simulink model "Regenerative_Braking"  (R2023a)
settings: Solver=ode23tb  StartTime=0.0  StopTime=300  MaxStep=0.1  MinStep=1e-4  RelTol=1e-2
values from neighbouring files (symbols this model uses):
  SOC = simOut.get('SOC')    [untitled.m]
undefined symbols (not defined in the file or in its folder): canChannel, T_cell
libraries: canmsglib x6, simulink x4, canlib x1
settings Model: Creator=MEHMET  LastModifiedBy=MEHMET
settings SolverCC: MaxConsecutiveMinStep=20
settings DebuggingCC: AlgebraicLoopMsg=none  ArtificialAlgebraicLoopMsg=none  ParameterPrecisionLossMsg=none  OperatingPointInterfaceChecksumMismatchMsg=none

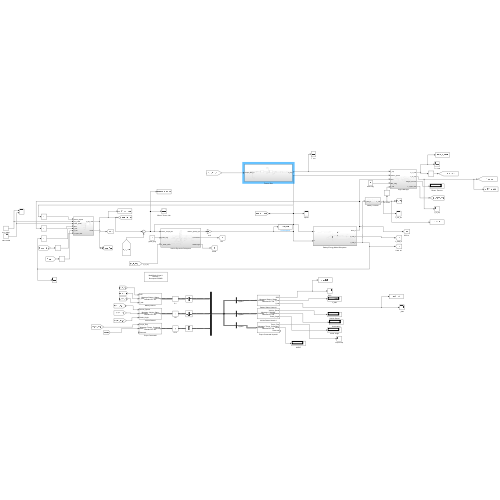
[thumbnail: Simulink's stored preview of the top-level diagram]
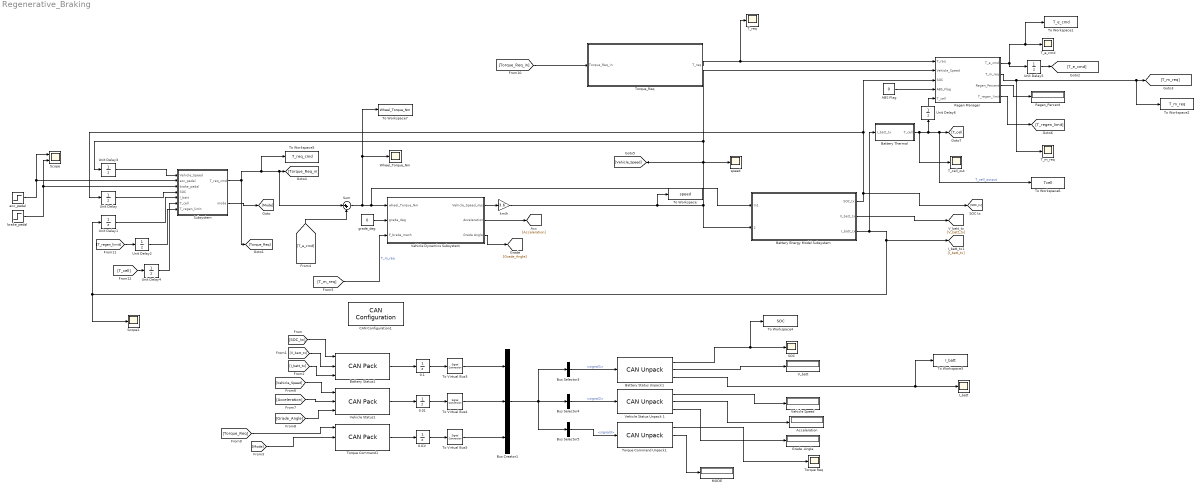
== system Regenerative_Braking ==
  0.01 : UnitDelay  InitialCondition=0.01  SampleTime=-1  HasFrameUpgradeWarning=on
  0.01! : UnitDelay  InitialCondition=0.1  SampleTime=-1  HasFrameUpgradeWarning=on
  0.1 : UnitDelay  InitialCondition=0.1  SampleTime=-1  HasFrameUpgradeWarning=on
  ABS Flag : Constant  Value=0
  Acceleration : Display
  Battery Energy Model Subsystem : Subsystem
  Battery Status Unpack1 : canmsglib/CAN Unpack  MsgList=(none)  MsgName=Battery_Status  MsgIDType=Standard (11-bit identifier)  MsgIdentifier=100  MsgLength=8  SignalInfo={ 'SOC', '0', '16', 'LE', 'signed', 'Standard', '0', '0.1', '0', '-Inf', 'Inf'; 'V_batt', '16', '16', 'LE', 'unsigned', 'Standard', '0', '0.1', '0', '-Inf', 'Inf'; 'I_batt', '32', '16', 'LE', 'signed', 'Standard', '0', '0.01', '0', '-Inf', 'Inf' }  IDPort=off  TimestampPort=off  ErrorPort=off  RemotePort=off  LengthPort=off  StatusPort=off  ApplyMinMax=off
      settings: LibrarySourceBlock=canlib/CAN Unpack
  Battery Status1 : canmsglib/CAN Pack  MsgList=(none)  MsgName=Battery_Status  MsgIDType=Standard (11-bit identifier)  MsgIdentifier=100  MsgLength=8  Remote=off  ApplyMinMax=off  BusOutput=on  SignalInfo={ 'SOC', '0', '16', 'LE', 'signed', 'Standard', '0', '0.1', '0', '-Inf', 'Inf'; 'V_batt', '16', '16', 'LE', 'unsigned', 'Standard', '0', '0.1', '0', '-Inf', 'Inf'; 'I_batt', '32', '16', 'LE', 'signed', 'Standard', '0', '0.01', '0', '-Inf', 'Inf' }
      settings: LibrarySourceBlock=canlib/CAN Pack  DataFormat=manually specified signals
  Battery Thermal : Subsystem
  Bus Creator1 : BusCreator  Inputs=3
  Bus Selector3 : BusSelector  OutputSignals=signal1
  Bus Selector4 : BusSelector  OutputSignals=signal2
  Bus Selector5 : BusSelector  OutputSignals=signal3
  CAN Configuration1 : canlib/CAN Configuration  BlockHandle=109.0284  Device=MathWorks Virtual 1 (Channel 1)  DeviceMenu=MathWorks Virtual 1 (Channel 1)  ObjConstructor=canChannel('MathWorks', 'Virtual 1', 1)  BusSpeed=500000  EnableBitParameters=off  AckMode=Normal
  Grade .Angle : Display
  I_batt : Scope
  MODE : Display
  Regen Manager : Subsystem
  Regen_Percent : Display
  SOC : Scope
  Scope : Scope  NumInputPorts=2
  Scope1 : Scope
  Subsystem : Subsystem
  Sum : Sum  Inputs=|++
  T_cell_out : Scope
  T_e_cmd : Scope
  T_m_req : Scope
  T_req : Scope
  To Virtual Bus3 : SignalConversion  ConversionOutput=Nonvirtual bus  OverrideOpt=off
  To Virtual Bus4 : SignalConversion  ConversionOutput=Nonvirtual bus  OverrideOpt=off
  To Virtual Bus5 : SignalConversion  ConversionOutput=Nonvirtual bus  OverrideOpt=off
  To Workspace : ToWorkspace  VariableName=speed  SampleTime=-1
  To Workspace1 : ToWorkspace  VariableName=T_e_cmd  SampleTime=-1
  To Workspace2 : ToWorkspace  VariableName=T_m_req  SampleTime=-1
  To Workspace3 : ToWorkspace  VariableName=I_batt  SampleTime=-1
  To Workspace4 : ToWorkspace  VariableName=SOC  SampleTime=-1
  To Workspace5 : ToWorkspace  VariableName=T_req_cmd  SampleTime=-1
  To Workspace6 : ToWorkspace  VariableName=Tcell  SampleTime=-1
  To Workspace7 : ToWorkspace  VariableName=Wheel_Torque_Nm  SampleTime=-1
  Torque Command Unpack1 : canmsglib/CAN Unpack  MsgList=(none)  MsgName=Torque_Command  MsgIDType=Standard (11-bit identifier)  MsgIdentifier=300  MsgLength=8  SignalInfo={ 'Torque_Req', '0', '32', 'LE', 'single', 'Standard', '0', '1', '0', '-Inf', 'Inf'; 'Mode', '32', '8', 'LE', 'unsigned', 'Standard', '0', '1', '0', '-Inf', 'Inf'; 'Reserved', '40', '8', 'LE', 'unsigned', 'Standard', '0', '1', '0', '-Inf', 'Inf' }  IDPort=off  TimestampPort=off  ErrorPort=off  RemotePort=off  LengthPort=off  StatusPort=off  ApplyMinMax=off
      settings: LibrarySourceBlock=canlib/CAN Unpack
  Torque Command1 : canmsglib/CAN Pack  MsgList=(none)  MsgName=Torque_Command  MsgIDType=Standard (11-bit identifier)  MsgIdentifier=300  MsgLength=8  Remote=off  ApplyMinMax=off  BusOutput=on  SignalInfo={ 'Torque_Req', '0', '32', 'LE', 'single', 'Standard', '0', '1', '0', '-Inf', 'Inf'; 'Mode', '32', '8', 'LE', 'unsigned', 'Standard', '0', '1', '0', '-Inf', 'Inf'; 'Reserved', '40', '8', 'LE', 'unsigned', 'Standard', '0', '1', '0', '-Inf', 'Inf' }
      settings: LibrarySourceBlock=canlib/CAN Pack  DataFormat=manually specified signals
  Torque Req : Scope
  Torque_Req : Subsystem
  Unit Delay{,1..5} (6 alike) : UnitDelay  SampleTime=0.01  HasFrameUpgradeWarning=on
  Unit Delay6 : UnitDelay  InitialCondition=0.01  SampleTime=-1  HasFrameUpgradeWarning=on
  V_batt : Display
  Vehicle Dynamics Subsystem : Subsystem
  Vehicle Speed : Display
  Vehicle Status Unpack 1 : canmsglib/CAN Unpack  MsgList=(none)  MsgName=CAN Msg  MsgIDType=Standard (11-bit identifier)  MsgIdentifier=200  MsgLength=8  SignalInfo={ 'Vehicle_Speed', '0', '16', 'LE', 'unsigned', 'Standard', '0', '0.1', '0', '-Inf', 'Inf'; 'Acceleration', '16', '16', 'LE', 'unsigned', 'Standard', '0', '0.01', '0', '-Inf', 'Inf'; 'Grade_Angle', '32', '16', 'LE', 'unsigned', 'Standard', '0', '0.1', '0', '-Inf', 'Inf' }  IDPort=off  TimestampPort=off  ErrorPort=off  RemotePort=off  LengthPort=off  StatusPort=off  ApplyMinMax=off
      settings: LibrarySourceBlock=canlib/CAN Unpack
  Vehicle Status1 : canmsglib/CAN Pack  MsgList=(none)  MsgName=Vehicle_State  MsgIDType=Standard (11-bit identifier)  MsgIdentifier=200  MsgLength=8  Remote=off  ApplyMinMax=off  BusOutput=on  SignalInfo={ 'Vehicle_Speed', '0', '16', 'LE', 'unsigned', 'Standard', '0', '0.1', '0', '-Inf', 'Inf'; 'Acceleration', '16', '16', 'LE', 'unsigned', 'Standard', '0', '0.01', '0', '-Inf', 'Inf'; 'Grade_Angle', '32', '16', 'LE', 'unsigned', 'Standard', '0', '0.1', '0', '-Inf', 'Inf' }
      settings: LibrarySourceBlock=canlib/CAN Pack  DataFormat=manually specified signals
  Wheel_Torque_Nm : Scope
  acc_pedal : Step  After=100  SampleTime=0  ZeroCross=off
  brake_pedal : Step  Time=100  After=300  SampleTime=0  ZeroCross=off
  grade_deg : Constant  Value=0
  km/h : Gain  Gain=3.6
  speed : Scope
  wires:
  Regen Manager/1(T_e_cmd) -> Unit Delay5/1, To Workspace1/1, T_e_cmd/1
  [Acceleration] -> Vehicle Status1/2
  Vehicle Status Unpack 1/2 -> Acceleration/1
  Vehicle Dynamics Subsystem/1(Vehicle_Speed_mps) -> km/h/1
  [Vehicle_Speed] -> Vehicle Status1/1
  Bus Creator1/1 -> Bus Selector5/1, Bus Selector3/1, Bus Selector4/1
  [Mode] -> Torque Command1/2
  Battery Status Unpack1/1 -> To Workspace4/1, SOC/1
  Battery Status Unpack1/3 -> To Workspace3/1, I_batt/1
  Battery Status Unpack1/2 -> V_batt/1
  [I_batt_tx] -> Battery Status1/3
  Bus Selector3/1 -> Battery Status Unpack1/1  "<signal1>"
  Vehicle Status Unpack 1/3 -> Grade .Angle/1
  Bus Selector4/1 -> Vehicle Status Unpack 1/1  "<signal2>"
  To Virtual Bus3/1 -> Bus Creator1/1
  Bus Selector5/1 -> Torque Command Unpack1/1  "<signal3>"
  Torque Command Unpack1/2 -> MODE/1
  Battery Status1/1 -> 0.1/1
  To Virtual Bus5/1 -> Bus Creator1/3
  Vehicle Dynamics Subsystem/3(Grade Angle) -> [Grade_Angle]
  To Virtual Bus4/1 -> Bus Creator1/2
  [V_batt_tx] -> Battery Status1/2
  Battery Energy Model Subsystem/2(V_batt_tx) -> [V_batt_tx]
  [SOC_tx] -> Battery Status1/1
  Vehicle Dynamics Subsystem/2(Acceleration) -> [Acceleration]
  [Grade_Angle] -> Vehicle Status1/3
  Regen Manager/3(Regen_Percent) -> Regen_Percent/1
  Torque Command1/1 -> 0.01!/1
  Regen Manager/2(T_m_req) -> T_m_req/1, To Workspace2/1, [T_m_req]
  grade_deg/1 -> Vehicle Dynamics Subsystem/2(grade_deg)
  0.01!/1 -> To Virtual Bus5/1
  ABS Flag/1 -> Regen Manager/4(ABS_Flag)
  Vehicle Status1/1 -> 0.01/1
  Torque Command Unpack1/1 -> Torque Req/1
  0.1/1 -> To Virtual Bus3/1
  Vehicle Status Unpack 1/1 -> Vehicle Speed/1
  Battery Energy Model Subsystem/3(I_batt_tx) -> Scope1/1, Unit Delay1/1, [I_batt_tx], Battery Thermal/1(I_batt_tx)
  [Torque_Req] -> Torque Command1/1
  Torque_Req/1(T_req) -> T_req/1, Regen Manager/1(T_req)
  0.01/1 -> To Virtual Bus4/1
  [Torque_Req_in] -> Torque_Req/1(Torque_Req_in)
  Sum/1 -> To Workspace7/1, Wheel_Torque_Nm/1, Battery Energy Model Subsystem/1(In1), Vehicle Dynamics Subsystem/1(wheel_Torque_Nm)
  [T_e_cmd] -> Sum/2
  [T_m_req] -> Vehicle Dynamics Subsystem/3(F_brake_mech)  "T_m_req"
  km/h/1 -> To Workspace/1, Unit Delay3/1, Regen Manager/2(Vehicle_Speed), speed/1, [Vehicle_Speed], Battery Energy Model Subsystem/2(2)
  Battery Energy Model Subsystem/1(SOC_tx) -> [SOC_tx], Regen Manager/3(SOC), Unit Delay/1
  Regen Manager/4(T_regen_limit) -> [T_regen_limit]
  Battery Thermal/1(T_cell) -> Unit Delay6/1, To Workspace6/1, [T_cell], T_cell_out/1  "T_cell_output"
  [T_regen_limit] -> Unit Delay2/1
  [T_cell] -> Unit Delay4/1
  Unit Delay5/1 -> [T_e_cmd]
  Unit Delay6/1 -> Regen Manager/5(T_cell)
  acc_pedal/1 -> Subsystem/2(acc_pedal), Scope/1
  brake_pedal/1 -> Subsystem/3(brake_pedal), Scope/2
  Unit Delay3/1 -> Subsystem/1(Vehicle_Speed)
  Unit Delay/1 -> Subsystem/4(SOC)
  Unit Delay1/1 -> Subsystem/5(I_batt)
  Unit Delay4/1 -> Subsystem/6(T_cell)
  Unit Delay2/1 -> Subsystem/7(T_regen_limit)
  Subsystem/1(T_req_cmd) -> To Workspace5/1, Sum/1, [Torque_Req_in], [Torque_Req]
  Subsystem/2(mode) -> [Mode]

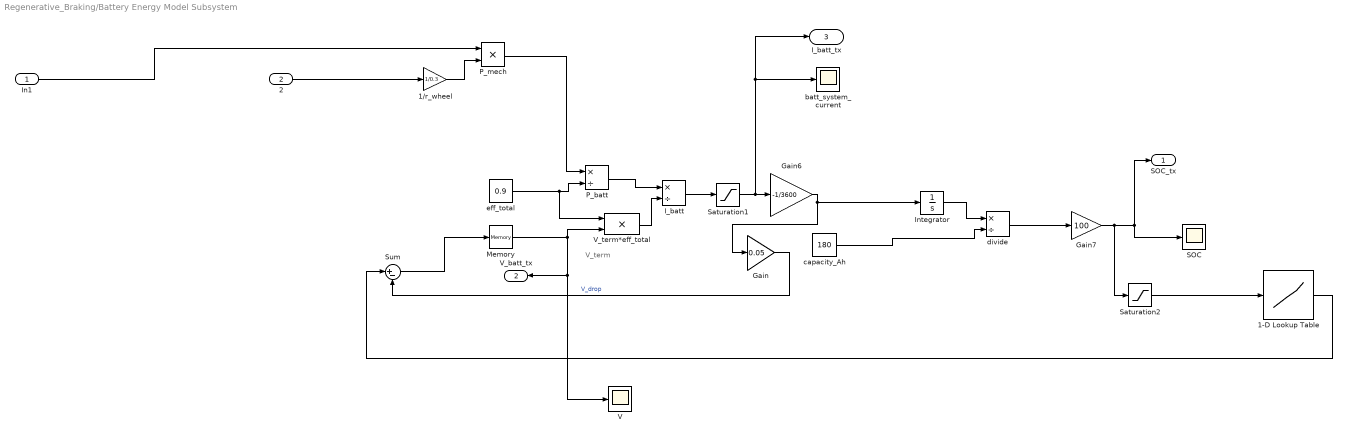
== system Regenerative_Braking/Battery Energy Model Subsystem ==
  note: V_term
  In1 : Inport
  2 : Inport  Port=2
  1-D Lookup Table : Lookup_n-D  NumberOfTableDimensions=1  BreakpointsForDimension1=[10 20 40 60 80 100]  Table=[325 332 342 350 356 360]  InternalRulePriority=Speed  RndMeth=Simplest
  1/r_wheel : Gain  Gain=1/0.3
  Gain : Gain  Gain=0.05
  Gain6 : Gain  Gain=-1/3600
  Gain7 : Gain  Gain=100
  I_batt : Product  Inputs=*/  RndMeth=Zero  SaturateOnIntegerOverflow=on
  Integrator : Integrator  InitialCondition=80  LimitOutput=on  UpperSaturationLimit=180  LowerSaturationLimit=0  ZeroCross=off
  Memory : Memory  InitialCondition=0.01
  P_batt : Product  Inputs=*/
  P_mech : Product
  SOC : Scope
  Saturation1 : Saturate  UpperLimit=300  LowerLimit=-300  ZeroCross=off
  Saturation2 : Saturate  UpperLimit=100  LowerLimit=0  ZeroCross=off
  Sum : Sum  Inputs=|+-
  V : Scope
  V_term*eff_total : Product
  batt_system_current : Scope
  capacity_Ah : Constant  Value=180
  divide : Product  Inputs=*/  RndMeth=Zero  SaturateOnIntegerOverflow=on
  eff_total : Constant  Value=0.9
  SOC_tx : Outport
  V_batt_tx : Outport  Port=2
  I_batt_tx : Outport  Port=3
  wires:
  P_batt/1 -> I_batt/1
  2/1 -> 1/r_wheel/1
  In1/1 -> P_mech/1
  capacity_Ah/1 -> divide/2
  1/r_wheel/1 -> P_mech/2
  P_mech/1 -> P_batt/1
  eff_total/1 -> V_term*eff_total/1, P_batt/2
  Gain7/1 -> Saturation2/1, SOC_tx/1, SOC/1
  1-D Lookup Table/1 -> Sum/1
  Memory/1 -> V/1, V_batt_tx/1, V_term*eff_total/2
  Sum/1 -> Memory/1
  Gain/1 -> Sum/2  "V_drop"
  V_term*eff_total/1 -> I_batt/2
  Integrator/1 -> divide/1
  I_batt/1 -> Saturation1/1
  Saturation1/1 -> I_batt_tx/1, batt_system_current/1, Gain6/1
  Saturation2/1 -> 1-D Lookup Table/1
  divide/1 -> Gain7/1
  Gain6/1 -> Integrator/1, Gain/1

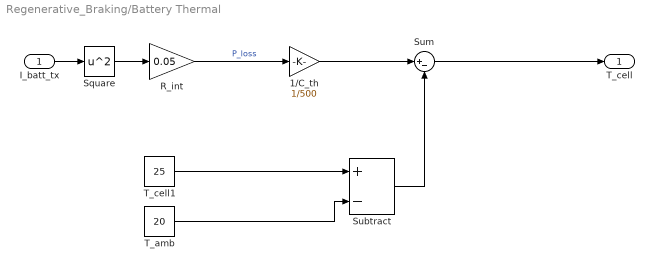
== system Regenerative_Braking/Battery Thermal ==
  I_batt_tx : Inport
  1/C_th : Gain  Gain=1/500
  R_int : Gain  Gain=0.05
  Square : Math  Operator=square
  Subtract : Sum  Inputs=+-
  Sum : Sum  Inputs=|+-
  T_amb : Constant  Value=20
  T_cell1 : Constant  Value=25
  T_cell : Outport
  wires:
  I_batt_tx/1 -> Square/1
  Square/1 -> R_int/1
  R_int/1 -> 1/C_th/1  "P_loss"
  1/C_th/1 -> Sum/1
  T_cell1/1 -> Subtract/1
  T_amb/1 -> Subtract/2
  Subtract/1 -> Sum/2
  Sum/1 -> T_cell/1

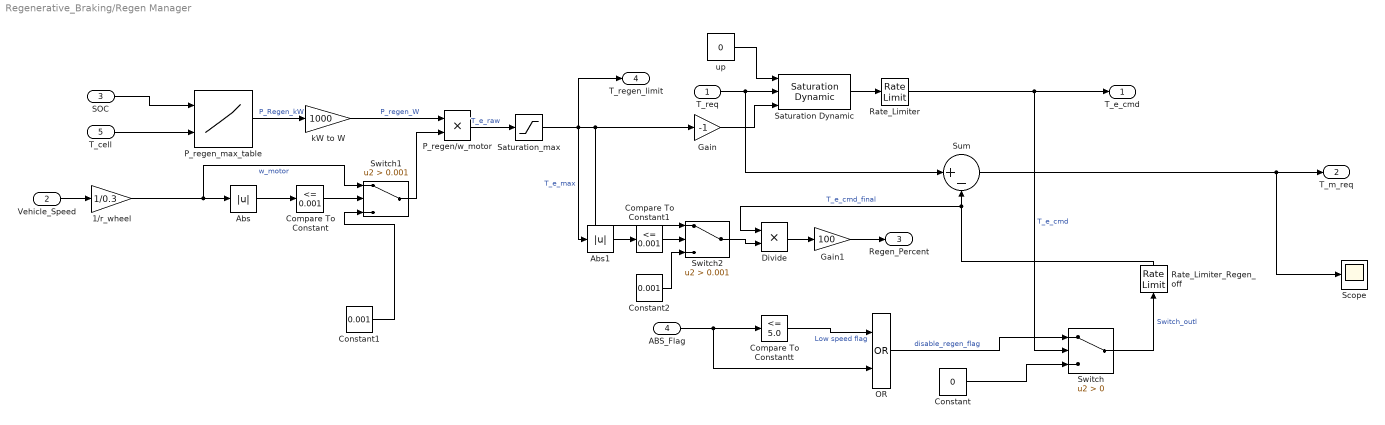
== system Regenerative_Braking/Regen Manager ==
  T_req : Inport
  Vehicle_Speed : Inport  Port=2
  SOC : Inport  Port=3
  ABS_Flag : Inport  Port=4
  T_cell : Inport  Port=5
  1/r_wheel : Gain  Gain=1/0.3
  Abs : Abs  ZeroCross=off  SaturateOnIntegerOverflow=off
  Abs1 : Abs  SaturateOnIntegerOverflow=off
  Compare To Constant : simulink/Logic and Bit Operations/Compare To Constant  relop=<=  const=0.001  OutDataTypeStr=boolean  ZeroCross=off
  Compare To Constant1 : simulink/Logic and Bit Operations/Compare To Constant  relop=<=  const=0.001  OutDataTypeStr=boolean  ZeroCross=off
  Compare To Constantt : simulink/Logic and Bit Operations/Compare To Constant  relop=<=  const=5.0  OutDataTypeStr=boolean  ZeroCross=off
  Constant : Constant  Value=0
  Constant1 : Constant  Value=0.001
  Constant2 : Constant  Value=0.001
  Divide : Product  RndMeth=Zero  SaturateOnIntegerOverflow=on
  Gain : Gain  Gain=-1
  Gain1 : Gain  Gain=100
  OR : Logic  Operator=OR  IconShape=distinctive  AllPortsSameDT=off  OutDataTypeStr=boolean
  P_regen/w_motor : Product  RndMeth=Zero  SaturateOnIntegerOverflow=on
  P_regen_max_table : Lookup_n-D  BreakpointsForDimension1=[0 20 40 60 80 95 100] % SOC  BreakpointsForDimension2="[-10 0 10 20 30 40 50]    % T_cell"  Table=|  InternalRulePriority=Speed  RndMeth=Simplest
      | [  5   10   15   20   25   20    0;
      |    8   15   25   35   45   35    0;
      |   12   30   45   60   70   50    0;
      |   15   40   60   80   90   60    0;
      |   15   40   60   80   90   60    0;
      |   10   30   45   60   70   50    0;
      |    5   15   25   35   45   35    0 ]
      settings: InputPortMap=u0,u1
  Rate_Limiter : RateLimiter  RisingSlewLimit=3000  FallingSlewLimit=-3000  SampleTimeMode=inherited
  Rate_Limiter_Regen_off : RateLimiter  RisingSlewLimit=2000  FallingSlewLimit=-2000  SampleTimeMode=inherited
  Saturation Dynamic : simulink/Discontinuities/Saturation Dynamic  OutMin=[]  OutMax=[]  OutDataTypeStr=Inherit: Same as second input  OutDataType=fixdt(1, 16)  OutScaling=2^-10  DoSatur=off
  Saturation_max : Saturate  UpperLimit=1500  LowerLimit=0  ZeroCross=off
  Scope : Scope
  Sum : Sum  Inputs=|+-
  Switch : Switch  Criteria=u2 > Threshold  SaturateOnIntegerOverflow=off  InputSameDT=off
  Switch1 : Switch  Criteria=u2 > Threshold  Threshold=0.001  SaturateOnIntegerOverflow=off  InputSameDT=off
  Switch2 : Switch  Criteria=u2 > Threshold  Threshold=0.001  SaturateOnIntegerOverflow=off  InputSameDT=off
  kW to W : Gain  Gain=1000
  up : Constant  Value=0
  T_e_cmd : Outport
  T_m_req : Outport  Port=2
  Regen_Percent : Outport  Port=3
  T_regen_limit : Outport  Port=4
  wires:
  SOC/1 -> P_regen_max_table/1
  T_cell/1 -> P_regen_max_table/2
  P_regen_max_table/1 -> kW to W/1  "P_Regen_kW"
  kW to W/1 -> P_regen/w_motor/1  "P_regen_W"
  Vehicle_Speed/1 -> 1/r_wheel/1
  1/r_wheel/1 -> Switch1/1, Abs/1  "w_motor"
  P_regen/w_motor/1 -> Saturation_max/1  "T_e_raw"
  Saturation_max/1 -> T_regen_limit/1, Abs1/1, Gain/1, Switch2/1  "T_e_max"
  T_req/1 -> Sum/1, Saturation Dynamic/2
  up/1 -> Saturation Dynamic/1
  Gain/1 -> Saturation Dynamic/3
  Saturation Dynamic/1 -> Rate_Limiter/1
  Rate_Limiter/1 -> Switch/2, T_e_cmd/1  "T_e_cmd"
  ABS_Flag/1 -> OR/2, Compare To Constantt/1
  Compare To Constantt/1 -> OR/1  "Low speed flag"
  OR/1 -> Switch/1  "disable_regen_flag"
  Constant/1 -> Switch/3
  Rate_Limiter_Regen_off/1 -> Divide/1, Sum/2  "T_e_cmd_final"
  Switch/1 -> Rate_Limiter_Regen_off/1  "Switch_outl"
  Divide/1 -> Gain1/1
  Gain1/1 -> Regen_Percent/1
  Abs/1 -> Compare To Constant/1
  Compare To Constant/1 -> Switch1/2
  Constant1/1 -> Switch1/3
  Switch1/1 -> P_regen/w_motor/2
  Abs1/1 -> Compare To Constant1/1
  Compare To Constant1/1 -> Switch2/2
  Switch2/1 -> Divide/2
  Constant2/1 -> Switch2/3
  Sum/1 -> Scope/1, T_m_req/1

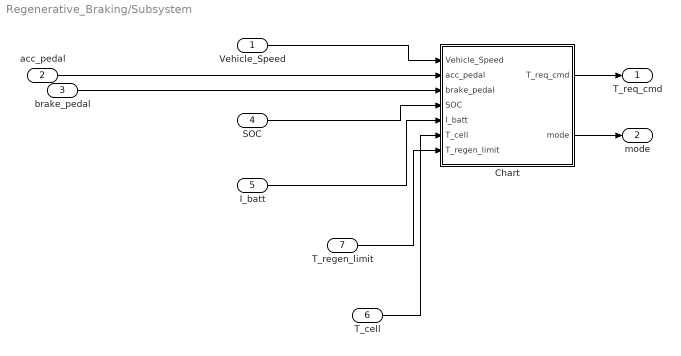
== system Regenerative_Braking/Subsystem ==
  Vehicle_Speed : Inport
  acc_pedal : Inport  Port=2
  brake_pedal : Inport  Port=3
  SOC : Inport  Port=4
  I_batt : Inport  Port=5
  T_cell : Inport  Port=6
  T_regen_limit : Inport  Port=7
  Chart : Stateflow chart  TreatAsAtomicUnit=on
  T_req_cmd : Outport
  mode : Outport  Port=2
  wires:
  Chart/2(mode) -> mode/1
  Chart/1(T_req_cmd) -> T_req_cmd/1
  T_cell/1 -> Chart/6(T_cell)
  Vehicle_Speed/1 -> Chart/1(Vehicle_Speed)
  acc_pedal/1 -> Chart/2(acc_pedal)
  I_batt/1 -> Chart/5(I_batt)
  SOC/1 -> Chart/4(SOC)
  T_regen_limit/1 -> Chart/7(T_regen_limit)
  brake_pedal/1 -> Chart/3(brake_pedal)

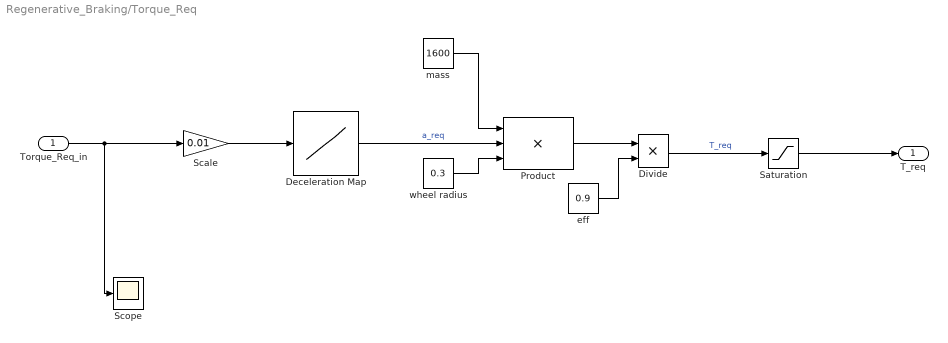
== system Regenerative_Braking/Torque_Req ==
  Torque_Req_in : Inport
  Deceleration Map : Lookup_n-D  NumberOfTableDimensions=1  BreakpointsForDimension1=[0 0.2 0.5 1.2 2.0 3.0 4.0]  Table=[0 10 20 40 60 80 100]  InternalRulePriority=Speed  RndMeth=Simplest
  Divide : Product  RndMeth=Zero  SaturateOnIntegerOverflow=on
  Product : Product  Inputs=3
  Saturation : Saturate  UpperLimit=300  LowerLimit=-300  ZeroCross=off
  Scale : Gain  Gain=0.01
  Scope : Scope
  eff : Constant  Value=0.9
  mass : Constant  Value=1600
  wheel radius : Constant  Value=0.3
  T_req : Outport
  wires:
  Scale/1 -> Deceleration Map/1
  Product/1 -> Divide/1
  wheel radius/1 -> Product/3
  Torque_Req_in/1 -> Scope/1, Scale/1
  mass/1 -> Product/1
  eff/1 -> Divide/2
  Deceleration Map/1 -> Product/2  "a_req"
  Divide/1 -> Saturation/1  "T_req"
  Saturation/1 -> T_req/1

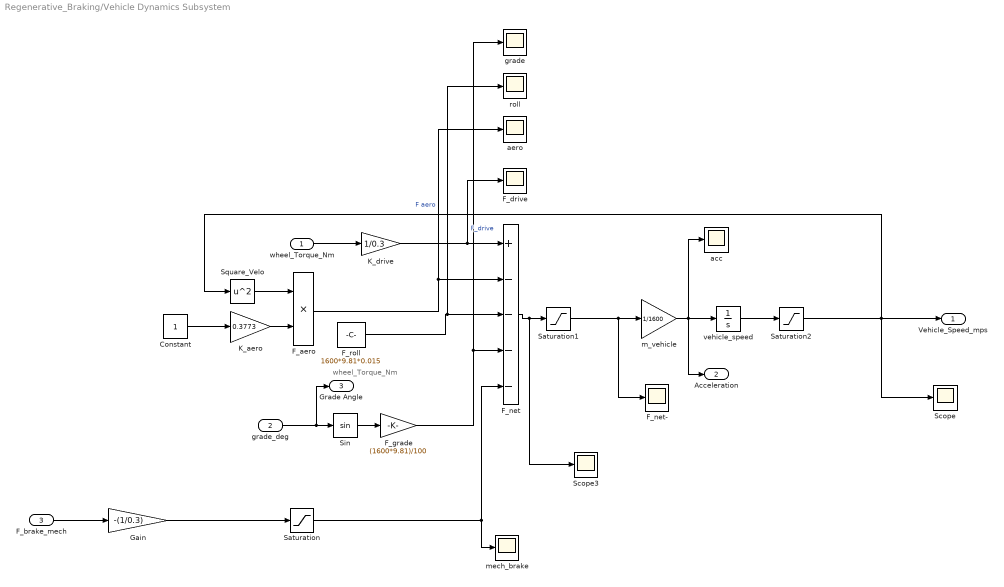
== system Regenerative_Braking/Vehicle Dynamics Subsystem ==
  note: wheel_Torque_Nm
  wheel_Torque_Nm : Inport
  grade_deg : Inport  Port=2
  F_brake_mech : Inport  Port=3
  Constant : Constant
  F_aero : Product
  F_drive : Scope
  F_grade : Gain  Gain=(1600*9.81)/100
  F_net : Sum  Inputs=+----
  F_net- : Scope
  F_roll : Constant  Value=1600*9.81*0.015
  Gain : Gain  Gain=-(1/0.3)
  K_aero : Gain  Gain=0.3773
  K_drive : Gain  Gain=1/0.3
  Saturation : Saturate  UpperLimit=10000  LowerLimit=0  ZeroCross=off
  Saturation1 : Saturate  UpperLimit=20000  LowerLimit=-20000  ZeroCross=off
  Saturation2 : Saturate  UpperLimit=50  LowerLimit=0  ZeroCross=off
  Scope : Scope
  Scope3 : Scope
  Sin : Trigonometry  OutputSignalType=real
  Square_Velo : Math  Operator=square
  acc : Scope
  aero : Scope
  grade : Scope
  m_vehicle : Gain  Gain=1/1600
  mech_brake : Scope
  roll : Scope
  vehicle_speed : Integrator  LimitOutput=on  UpperSaturationLimit=50  LowerSaturationLimit=0  ZeroCross=off
  Vehicle_Speed_mps : Outport
  Acceleration : Outport  Port=2
  Grade Angle : Outport  Port=3
  wires:
  Square_Velo/1 -> F_aero/1
  F_grade/1 -> grade/1, F_net/4
  K_drive/1 -> F_drive/1, F_net/1  "F_drive"
  F_aero/1 -> aero/1, F_net/2  "F aero"
  F_roll/1 -> roll/1, F_net/3
  Constant/1 -> K_aero/1
  K_aero/1 -> F_aero/2
  wheel_Torque_Nm/1 -> K_drive/1
  F_brake_mech/1 -> Gain/1
  grade_deg/1 -> Sin/1, Grade Angle/1
  Sin/1 -> F_grade/1
  F_net/1 -> Saturation1/1, Scope3/1
  Saturation/1 -> mech_brake/1, F_net/5
  Gain/1 -> Saturation/1
  Saturation1/1 -> F_net-/1, m_vehicle/1
  m_vehicle/1 -> vehicle_speed/1, acc/1, Acceleration/1
  vehicle_speed/1 -> Saturation2/1
  Saturation2/1 -> Scope/1, Vehicle_Speed_mps/1, Square_Velo/1

== stateflow chart Regenerative_Braking/Subsystem/Chart ==
  state Braking_State__
    entry:
    mode = 2;
    during:
    %==================================================
    % 1) SOC tabanlı regen limiti
    %==================================================
    if SOC > 85
    regen_limit = 0;          % SOC çok yüksek -> regen yok
    elseif SOC > 70
    regen_limit = -40;        % orta SOC -> sınırlı regen
    else
    regen_limit = -80;        % düşük SOC -> tam regen
    end
    %==================================================
    % 2) Hız tabanlı güvenlik limiti
    %==================================================
    if Vehicle_Speed > 10
    T_target = regen_limit;       % yüksek hız -> tam seçilen regen
    elseif Vehicle_Speed > 3
    T_target = regen_limit / 2;   % yavaşlarken -> daha hafif regen
    else
    T_target = 0;                 % durmaya yakın -> regen kapalı
    end
    %==================================================
    % 3) Akım koruma (charge current limit)
    %   Senin modelinde regen sırasında I_batt negatife düşüyorsa
    %   I_chg_max'i negatif tanımlayıp bu kıyaslama mantıklı olur.
    %==================================================
    if I_batt < I_chg_max
    % şarj akımı çok arttı -> regen torkunu azalt
    T_target = T_target * 0.7;
    end
    %==================================================
    % 4) Sıcaklık koruma
    %==================================================
    if T_cell > T_hot
    % Batarya fazla sıcak -> regen tamamen kapalı
    T_target = 0;
    elseif T_cell > T_warm
    % Ilık/sıcak aralık -> regen torkunu yarıya düşür
    T_target = T_target * 0.5;
    end
    % Çıkış tork komutu
    T_req_cmd = T_target;
  state Idle_
    entry:
    mode = 0;
    target_T = 0;
    T_req_cmd =0;
  state Drive_State__
    entry:
    mode = 1;
    T_target = acc_pedal * 10;   % 100 pedal -> 1000 Nm gibi
    during:
    %--------------------------------------------------
    % 1) SOC koruma
    %--------------------------------------------------
    if SOC < SOC_min
    T_limit = 100;           % SOC çok düşük -> tork sınırı 100 Nm
    else
    T_limit = T_max;         % normal limit
    end
    %--------------------------------------------------
    % 2) Akım koruma (decharge current limit)
    %   Pozitif akım = motora güç veriyoruz
    %--------------------------------------------------
    if I_batt > I_dis_max
    T_target = T_target * 0.7;   % çekiş torkunu azalt -> bataryayı koru
    end
    %--------------------------------------------------
    % 3) Sıcaklık koruma
    %   Batarya ısındıkça torku kıs
    %--------------------------------------------------
    if T_cell > T_hot
    % Çok sıcak -> çekişi kes
    T_target = 0;
    elseif T_cell > T_warm
    % Ilık/sıcak aralık -> torku %50 düşür
    T_target = T_target * 0.5;
    end
    %--------------------------------------------------
    % 4) Son tork limiti uygula
    %--------------------------------------------------
    T_target = min(T_target, T_limit);
    % ECU çıkışı
    T_req_cmd = T_target;
  Drive_State__ -> Braking_State__ [order 2] : [brake_pedal > 5]
  (default) -> Idle_
  Idle_ -> Drive_State__ : [acc_pedal > 50 && brake_pedal < 3]
  Drive_State__ -> Idle_ [order 1] : [acc_pedal < 3 && brake_pedal < 3]
  Braking_State__ -> Drive_State__ : [acc_pedal > 50 && brake_pedal < 3]
  data: T_req_cmd output double size=1 =0; mode output size=1; Vehicle_Speed input double size=1; T_target local double size=1 =0; acc_pedal input double size=1; brake_pedal input double size=1; SOC input size=1; regen_limit local size=1; I_batt input double size=1; T_max constant double =300; I_chg_max constant double =-200; target_T local; T_limit local; I_dis_max constant double =300; SOC_min constant double =30; T_cell input double size=1; T_warm constant double =35; T_hot constant double =45; T_regen_limit input size=1
  data mode settings: description=ECU operating mode (0=Idle, 1=Accel, 2=Cruise, 3=Decel
